simulink model "trafficlight"  (R2020b)
settings: Solver=VariableStepAuto  StartTime=0.0  StopTime=10.0  RelTol=1e-3
undefined symbols (not defined in the file): DiscIntNeverNeededParam
libraries: simulink x1
settings Model: Creator=sonal  LastModifiedBy=sonal

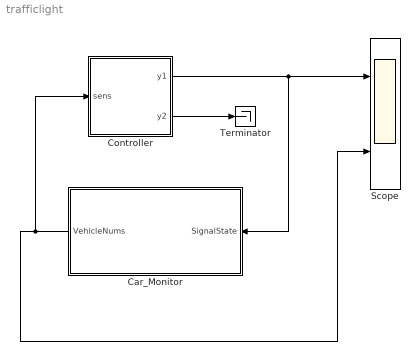
== system trafficlight ==
  Car_Monitor : Subsystem
  Controller : Stateflow chart  TreatAsAtomicUnit=on
  Scope : Scope  NumInputPorts=2
  Terminator : Terminator
  wires:
  Controller/2(y2) -> Terminator/1
  Controller/1(y1) -> Car_Monitor/1(SignalState), Scope/1
  Car_Monitor/1(VehicleNums) -> Controller/1(sens), Scope/2

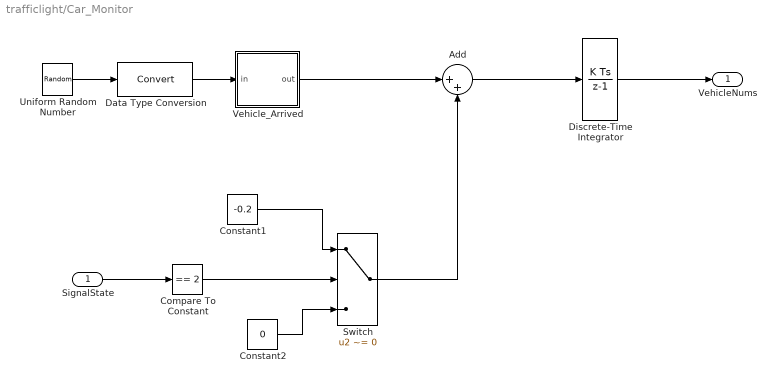
== system trafficlight/Car_Monitor ==
  SignalState : Inport
  Add : Sum  Inputs=|++
  Compare To Constant : simulink/Logic and Bit Operations/Compare To Constant  relop===  const=2  OutDataTypeStr=boolean  ZeroCross=off
  Constant1 : Constant  Value=-0.2
  Constant2 : Constant  Value=0
  Data Type Conversion : DataTypeConversion
  Discrete-Time Integrator : DiscreteIntegrator  SampleTime=-1  LimitOutput=on  LowerSaturationLimit=0  ICPrevOutput=DiscIntNeverNeededParam  ICPrevScaledInput=DiscIntNeverNeededParam
  Switch : Switch  Criteria=u2 ~= 0
  Uniform Random Number : UniformRandomNumber  Minimum=0  Maximum=100  Seed=177836  SampleTime=0
  Vehicle_Arrived : Stateflow chart  TreatAsAtomicUnit=on
  VehicleNums : Outport  VectorParamsAs1DForOutWhenUnconnected=off
  wires:
  Constant1/1 -> Switch/1
  Constant2/1 -> Switch/3
  Discrete-Time Integrator/1 -> VehicleNums/1
  SignalState/1 -> Compare To Constant/1
  Compare To Constant/1 -> Switch/2
  Switch/1 -> Add/2
  Add/1 -> Discrete-Time Integrator/1
  Vehicle_Arrived/1(out) -> Add/1
  Data Type Conversion/1 -> Vehicle_Arrived/1(in)
  Uniform Random Number/1 -> Data Type Conversion/1

== stateflow chart trafficlight/Controller ==
  settings: stateMachineType=MOORE_MACHINE
  state Stop
    y1 = Red;
    y2 = Green;
  state StopForTraffic
    y1 = Red;
    y2 = Green;
  state StopToGo
    y1 = Red;
    y2 = Yellow;
  state GoToStop
    y1 = Yellow;
    y2 = Red;
  state Go
    y1 = Green;
    y2 = Red;
  (default) -> Stop
  StopForTraffic -> StopToGo : [sens]
  Stop -> StopForTraffic : after(20,tick)
  GoToStop -> Stop : after (3,tick)
  StopToGo -> Go : after(3,tick)
  Go -> GoToStop : after(10,tick)
  data: sens input; y1 output; y2 output; Green constant double =1; Red constant double =3; Yellow constant double =2

== stateflow chart trafficlight/Car_Monitor/Vehicle_Arrived ==
  (default) -> (junction 2) : {out = in > 98;}
  data: in input int8; out output double
